simulink model "ESKF"  (R2024a)
settings: Solver=VariableStepAuto  StartTime=0.0  StopTime=10.0  RelTol=1e-3
undefined symbols (not defined in the file): dt_imu, g_n, R_pos, R_vel, sigma_acc, sigma_ba, sigma_bg, sigma_gyr
libraries: simulink x1
settings Model: DataDictionary=StateEstDict.sldd  Creator=89447  LastModifiedBy=89447

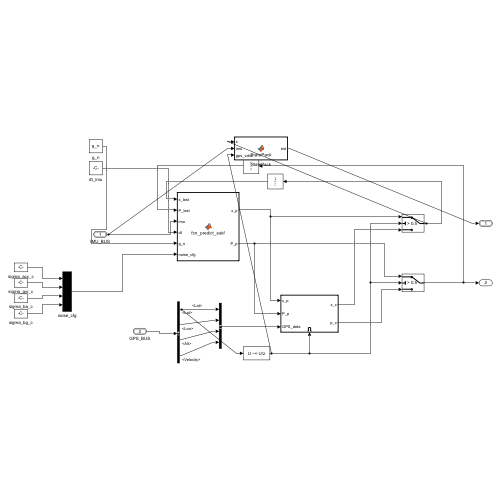
[thumbnail: Simulink's stored preview of the top-level diagram]
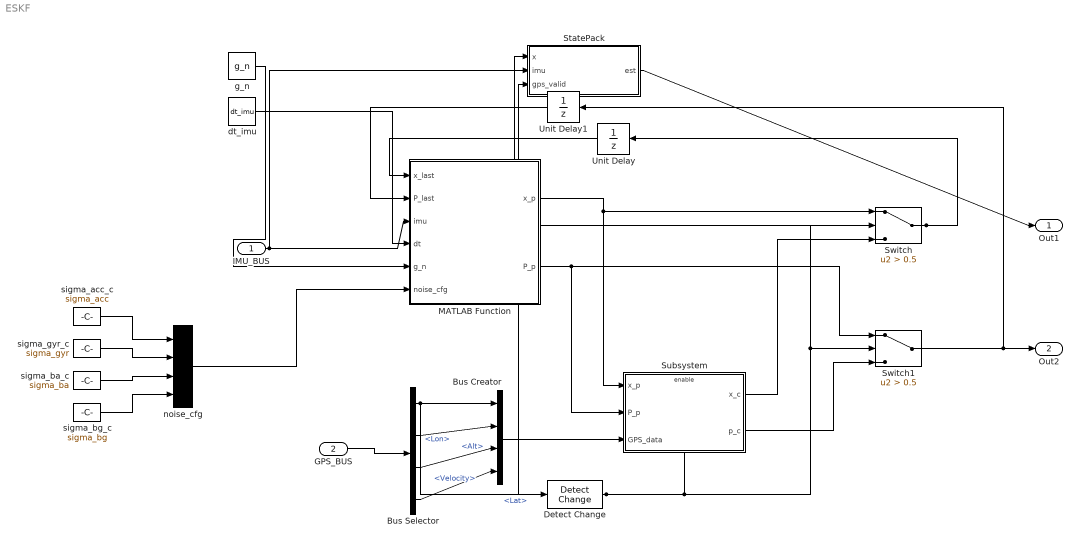
== system ESKF ==
  IMU_BUS : Inport  OutDataTypeStr=Bus: IMU_BUS
  GPS_BUS : Inport  Port=2  OutDataTypeStr=Bus: GPS_BUS
  Bus Creator : BusCreator  Inputs=4
  Bus Selector : BusSelector  OutputSignals=Lat,Lon,Alt,Velocity
  Detect Change : simulink/Logic and Bit Operations/Detect Change  vinit=0  OutDataTypeStr=boolean
  MATLAB Function : MATLAB Function  TreatAsAtomicUnit=on
  StatePack : MATLAB Function  TreatAsAtomicUnit=on
  Subsystem : Subsystem
  Switch : Switch  Criteria=u2 > Threshold  Threshold=0.5  SaturateOnIntegerOverflow=off  InputSameDT=off
  Switch1 : Switch  Criteria=u2 > Threshold  Threshold=0.5  SaturateOnIntegerOverflow=off  InputSameDT=off
  Unit Delay : UnitDelay  InitialCondition=[0;0;0;0;0;0;1;0;0;0;0;0;0;0;0;0]  SampleTime=-1  HasFrameUpgradeWarning=on
  Unit Delay1 : UnitDelay  InitialCondition=[1 0 0 0 0 0 0 0 0 0 0 0 0 0 0;0 1 0 0 0 0 0 0 0 0 0 0 0 0 0;0 0 1 0 0 0 0 0 0 0 0 0 0 0 0;0 0 0 1 0 0 0 0 0 0 0 0 0 0 0;0 0 0 0 1 0 0 0 0 0 0 0 0 0 0;0 0 0 0 0 1 0 0 0 0 0 0 0 0 0;0 0 0 0 0 0 0.100000001490116 0 0 0 0 0 0 0 0;0 0 0 0 0 0 0 0.100000001490116 0 0 0 0 0 0 0;0 0 0 0 0 0 0 0 0.100000001490116 0 0 0 0 0 0;0 0 0 0 0 0 0 0 0 0.00999999977648258 0 0 0 0 0;0 0 0 0 0 0 0 0 0 0 0.00999999977648258 0 0 0 0;0 0 0 0 0 0 0 0 0 0 0 0.00999999977648258 0 0 0;0 0 0 0 0 0 0 0 0 0 0 0 0.00999999977648258 0 0;0 0 0 0 0 0 0 0 0 0 0 0 0 0.00999999977648258 0;0 0 0 0 0 0 0 0 0 0 0 0 0 0 0.00999999977648258]  SampleTime=-1  HasFrameUpgradeWarning=on
  dt_imu : Constant  Value=dt_imu  OutDataTypeStr=single
  g_n : Constant  Value=g_n  OutDataTypeStr=single
  noise_cfg : Mux
  sigma_acc_c : Constant  Value=sigma_acc  OutDataTypeStr=single
  sigma_ba_c : Constant  Value=sigma_ba  OutDataTypeStr=single
  sigma_bg_c : Constant  Value=sigma_bg  OutDataTypeStr=single
  sigma_gyr_c : Constant  Value=sigma_gyr  OutDataTypeStr=single
  Out1 : Outport  OutDataTypeStr=Bus: StateEstBus
  Out2 : Outport  Port=2
  wires:
  MATLAB Function/1(x_p) -> Switch/1, Subsystem/1(x_p)
  IMU_BUS/1 -> MATLAB Function/3(imu), StatePack/2(imu)
  Bus Creator/1 -> Subsystem/3(GPS_data)
  Detect Change/1 -> Subsystem/Enable, Switch/2, Switch1/2, StatePack/3(gps_valid)
  Unit Delay/1 -> MATLAB Function/1(x_last)
  MATLAB Function/2(P_p) -> Subsystem/2(P_p), Switch1/1
  Switch/1 -> Unit Delay/1, StatePack/1(x)
  Subsystem/1(x_c) -> Switch/3
  Unit Delay1/1 -> MATLAB Function/2(P_last)
  Subsystem/2(p_c) -> Switch1/3
  Switch1/1 -> Unit Delay1/1, Out2/1
  GPS_BUS/1 -> Bus Selector/1
  sigma_acc_c/1 -> noise_cfg/1
  sigma_gyr_c/1 -> noise_cfg/2
  sigma_ba_c/1 -> noise_cfg/3
  sigma_bg_c/1 -> noise_cfg/4
  g_n/1 -> MATLAB Function/5(g_n)
  dt_imu/1 -> MATLAB Function/4(dt)
  noise_cfg/1 -> MATLAB Function/6(noise_cfg)
  Bus Selector/1 -> Bus Creator/1, Detect Change/1  "<Lat>"
  Bus Selector/2 -> Bus Creator/2  "<Lon>"
  Bus Selector/3 -> Bus Creator/3  "<Alt>"
  Bus Selector/4 -> Bus Creator/4  "<Velocity>"
  StatePack/1(est) -> Out1/1

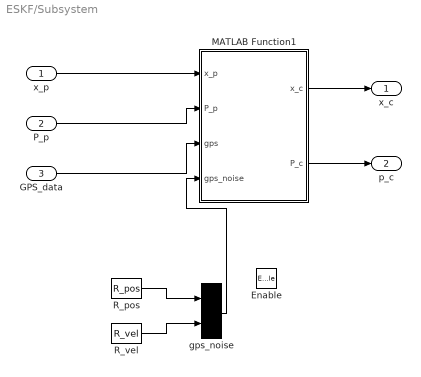
== system ESKF/Subsystem ==
  x_p : Inport
  P_p : Inport  Port=2
  GPS_data : Inport  Port=3
  Enable : EnablePort
  MATLAB Function1 : MATLAB Function  TreatAsAtomicUnit=on
  R_pos : Constant  Value=R_pos  OutDataTypeStr=single
  R_vel : Constant  Value=R_vel  OutDataTypeStr=single
  gps_noise : Mux  Inputs=2
  x_c : Outport
  p_c : Outport  Port=2
  wires:
  MATLAB Function1/1(x_c) -> x_c/1
  GPS_data/1 -> MATLAB Function1/3(gps)
  x_p/1 -> MATLAB Function1/1(x_p)
  P_p/1 -> MATLAB Function1/2(P_p)
  MATLAB Function1/2(P_c) -> p_c/1
  R_pos/1 -> gps_noise/1
  R_vel/1 -> gps_noise/2
  gps_noise/1 -> MATLAB Function1/4(gps_noise)

== matlab function ESKF/StatePack ==
  data: x input; est output Bus: StateEstBus; imu input; gps_valid input
function est = StatePack(x, imu, gps_valid)
%#codegen
% x(16x1): [p;v;q;ba;bg]
est.Position_NED     = single(x(1:3));
est.Velocity_NED     = single(x(4:6));
est.Attitude_quat    = single(x(7:10));
est.AngularRate_Body = single(imu.Gyro - x(14:16));
est.Accel_Body       = single(imu.Accel - x(11:13));
est.GyroBias         = single(x(14:16));
est.AccelBias        = single(x(11:13));
est.Wind_NED         = single([0;0;0]);
est.Status           = uint8(gps_valid);
end

== matlab function ESKF/MATLAB Function ==
  data: x_last input single size=16; x_p output single size=16; P_last input single size=[15, 15]; imu input Bus: IMU_BUS; P_p output single size=[15, 15]; dt input single size=1; g_n input single size=3; noise_cfg input single size=4
function [x_p, P_p] = fcn_predict_eskf(x_last, P_last, imu, dt, g_n, noise_cfg)
%#codegen
sigma_acc = noise_cfg(1);
sigma_gyr = noise_cfg(2);
sigma_ba  = noise_cfg(3);
sigma_bg  = noise_cfg(4);
Q_c = diag([sigma_acc*ones(1,3), sigma_gyr*ones(1,3), sigma_ba*ones(1,3), sigma_bg*ones(1,3)]);
p = x_last(1:3);
v = x_last(4:6);
q = x_last(7:10);
ba = x_last(11:13);
bg = x_last(14:16);
accel_corr = imu.Accel - ba;
omega_corr = imu.Gyro - bg;
dq = quat_exp(omega_corr, dt);
q_p = quat_mult(q, dq);
q_p = quat_normalize(q_p);
C_bn = quat2rotm(q);
a_n = C_bn * accel_corr + g_n;
v_p = v + a_n * dt;
p_p = p + v * dt + 0.5 * a_n * dt^2;
x_p = [p_p; v_p; q_p; ba; bg];
F_c = zeros(15, 15);
a_sk = skew_sym(accel_corr);
w_sk = skew_sym(omega_corr);
F_c(1:3, 4:6)   = eye(3);
F_c(4:6, 7:9)   = -C_bn * a_sk;
F_c(4:6, 10:12) = -C_bn;
F_c(7:9, 7:9)   = -w_sk;
F_c(7:9, 13:15) = -eye(3);
F = eye(15) + F_c * dt;
G = zeros(15, 12);
G(4:6, 1:3)   = -C_bn;
G(7:9, 4:6)   = -eye(3);
G(10:12, 7:9) = eye(3);
G(13:15, 10:12)= eye(3);
Q_d = G * Q_c * G' * dt;
P_p = F * P_last * F' + Q_d;
P_p = (P_p + P_p') / 2;
end

== matlab function ESKF/Subsystem/MATLAB Function1 ==
  data: x_p input single size=16; x_c output single size=16; P_p input single size=[15, 15]; gps input Bus: GPS_BUS; P_c output single size=[15, 15]; gps_noise input single size=2
function [x_c, P_c] = fcn_update(x_p, P_p, gps, gps_noise)
%#codegen
R_pos = gps_noise(1);
R_vel = gps_noise(2);
z = [gps.Lat; gps.Lon; gps.Alt; gps.Velocity];
H = zeros(6, 15);
H(1:3, 1:3) = eye(3);
H(4:6, 4:6) = eye(3);
R = diag([R_pos*ones(1,3), R_vel*ones(1,3)]);
S = H * P_p * H' + R;
K = (P_p * H') / S;
innovation = z - [x_p(1:3); x_p(4:6)];
dx = K * innovation;
x_c = x_p;
x_c(1:3)  = x_p(1:3)  + dx(1:3);
x_c(4:6)  = x_p(4:6)  + dx(4:6);
dq = quat_exp(dx(7:9), single(1.0));
x_c(7:10) = quat_mult(dq, x_p(7:10));
x_c(7:10) = quat_normalize(x_c(7:10));
x_c(11:13) = x_p(11:13) + dx(10:12);
x_c(14:16) = x_p(14:16) + dx(13:15);
I15 = eye(15);
P_c = (I15 - K*H) * P_p * (I15 - K*H)' + K * R * K';
P_c = (P_c + P_c') / 2;
end
